simulink model "Exercise_30"  (R2023a)
settings: Solver=VariableStepAuto  StartTime=0.0  StopTime=10.0  RelTol=1e-3
settings Model: Creator=Admin  LastModifiedBy=Admin

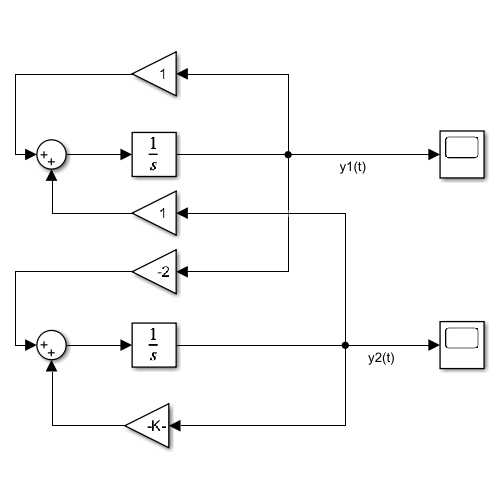
[thumbnail: Simulink's stored preview of the top-level diagram]
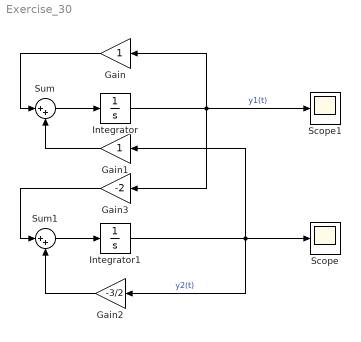
== system Exercise_30 ==
  Gain : Gain
  Gain1 : Gain
  Gain2 : Gain  Gain=-3/2
  Gain3 : Gain  Gain=-2
  Integrator : Integrator  InitialCondition=1
  Integrator1 : Integrator  InitialCondition=1
  Scope : Scope
  Scope1 : Scope
  Sum : Sum  Inputs=|++
  Sum1 : Sum  Inputs=|++
  wires:
  Integrator/1 -> Gain3/1, Gain/1, Scope1/1  "y1(t)"
  Integrator1/1 -> Gain2/1, Gain1/1, Scope/1  "y2(t)"
  Gain/1 -> Sum/1
  Sum/1 -> Integrator/1
  Gain1/1 -> Sum/2
  Gain3/1 -> Sum1/1
  Gain2/1 -> Sum1/2
  Sum1/1 -> Integrator1/1
